simulink model "sigmadelta_full_DCO_Sampled_differential_integer_true"  (R2023b)
settings: Solver=VariableStepAuto  StartTime=0.0  StopTime=(lsim+10)*Ts  RelTol=1e-9
values from neighbouring files (symbols this model uses):
  f0 = fs*NC1/32    (= 98304000)    [exe_sigmadelta_full_DCO_differential_integer_true.m]
  f02 = f0    (= 98304000)    [exe_sigmadelta_full_DCO_differential_integer_true.m]
  ft = (bint-1)*fbin    [exe_sigmadelta_full_DCO_differential_integer_true.m]
  Input_signal = 10^(Input_signal_dB/20)    (= 0.24831331053)    [exe_sigmadelta_full_DCO_differential_integer_true.m]
  Kvco = f0*1    (= 98304000)    [exe_sigmadelta_full_DCO_differential_integer_true.m]
  NbC1 = Nbvco+Nbext    (= 10)    [exe_sigmadelta_full_DCO_differential_integer_true.m]
  Nbdcoext = 3    [exe_sigmadelta_full_DCO_differential_integer_true.m]
  T2 = 1/f2    (= 4.06901041667e-08)    [exe_sigmadelta_full_DCO_differential_integer_true.m]
  Ts = 1/fs    (= 3.25520833333e-07)    [exe_sigmadelta_full_DCO_differential_integer_true.m]
libraries: dspsigops x4
settings Model: SimulationMode=accelerator  ExtModeTrigDuration=100  Creator=user  LastModifiedBy=Richi
settings SolverCC: AlgebraicLoopSolver=TrustRegion
settings DataIOCC: SaveFinalState=on  SaveFormat=Array  SaveOutput=off  SaveState=on  ReturnWorkspaceOutputs=off  StateSaveName=tmp_raccel_xout  SignalLoggingName=tmp_raccel_logsout
settings OptimizationCC: BlockReduction=off  BooleanDataType=off  ReuseModelBlockBuffer=off  EfficientMapNaN2IntZero=off  LifeSpan=inf
settings DebuggingCC: SaveWithParameterizedLinksMsg=none  UnderspecifiedInitializationDetection=Classic  MergeDetectMultiDrivingBlocksExec=none  SignalResolutionControl=TryResolveAllWithWarning  MultiTaskDSMMsg=warning  MultiTaskCondExecSysMsg=none  UnconnectedInputMsg=warning  UnconnectedOutputMsg=warning  UnconnectedLineMsg=warning  SFUnexpectedBacktrackingDiag=warning  SFNoUnconditionalDefaultTransitionDiag=warning  SFExecutionAtInitializationDiag=none  ArithmeticOperatorsInVariantConditions=warning
settings HardwareCC: ProdBitPerPointer=32  ProdBitPerSizeT=32  ProdBitPerPtrDiffT=32  ProdLargestAtomicFloat=None  ProdIntDivRoundTo=Undefined  ProdEndianess=Unspecified  ProdWordSize=32  ProdHWDeviceType=32-bit Generic  TargetBitPerPointer=64  TargetBitPerSizeT=64  TargetBitPerPtrDiffT=64  TargetLongLongMode=on  TargetIntDivRoundTo=Zero  TargetEndianess=LittleEndian  TargetWordSize=64  TargetHWDeviceType=MATLAB Host  ProdEqTarget=off
settings ModelReferenceCC: EnableRefExpFcnMdlSchedulingChecks=on  PropagateSignalLabelsOutOfModel=off
settings SFSimCC: SimUseLocalCustomCode=off  CustomCodeUndefinedFunction=UseInterfaceOnly
settings RTWCC: SystemTargetFile=raccel.tlc  TemplateMakefile=raccel_default_tmf  RTWVerbose=off  RTWUseLocalCustomCode=off  RTWUseSimCustomCode=on  DLArmComputeVersion=19.05
settings CodeAppCC: GenerateComments=off  MaxIdLength=128  MangleLength=10  SimulinkBlockComments=off
settings RaccelTargetCC: ParMdlRefBuildCompliant=off  OptimizeReductions=off  ENABLE_SLEXEC_SSBRIDGE=0  RTWCAPISignals=off  RTWCAPIParams=off  RTWCAPIRootIO=off
settings ConfigComp: CovMetricSettings=dw  CovSaveCumulativeToWorkspaceVar=on  CovSaveSingleToWorkspaceVar=on  CovExternalEMLEnable=off

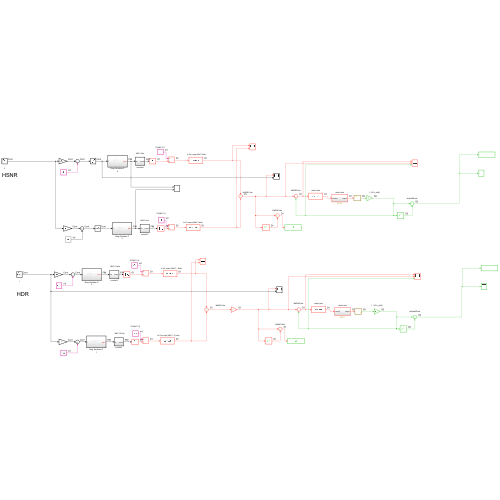
[thumbnail: Simulink's stored preview of the top-level diagram]
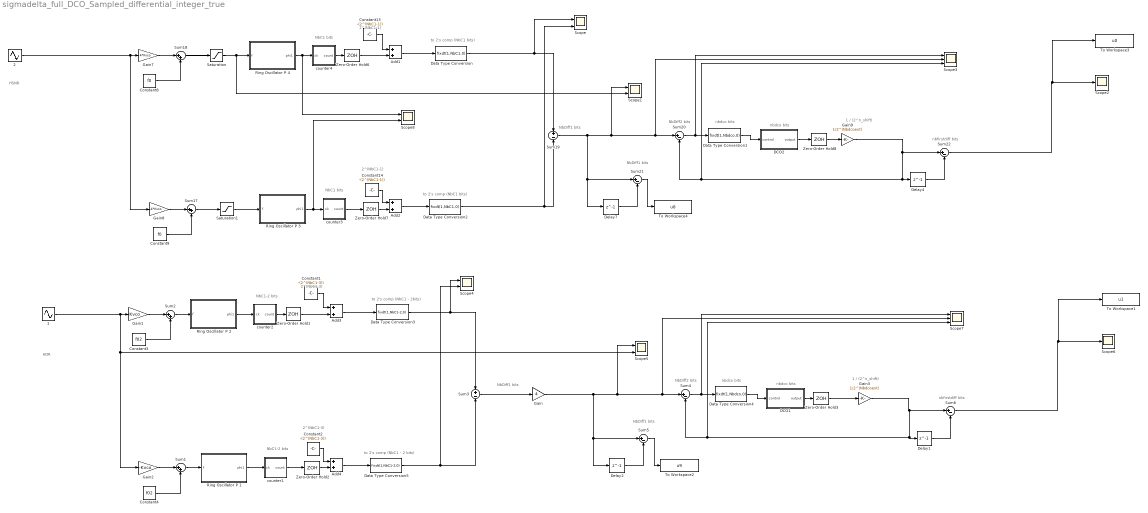
== system sigmadelta_full_DCO_Sampled_differential_integer_true ==
  note: HSNR
  note: nbfirstdiff bits
  note: 1 / (2^n_shift)
  note: nbdco bits
  note: NbDiff2 bits
  note: nbdco bits
  note: NbDiff1 bits
  note: 2^(NbC1-1)
  note: NbC1 bits
  note: NbC1 bits
  note: 2^(NbC1-1)
  note: to 2's comp (NbC1 bits)
  note: to 2's comp (NbC1 bits)
  note: NbDiff1 bits
  note: nbfirstdiff bits
  note: 1 / (2^n_shift)
  note: NbDiff1 bits
  note: to 2's comp (NbC1 - 2 bits)
  note: NbC1-2 bits
  note: nbdco bits
  note: NbDiff1 bits
  note: to 2's comp (NbC1 - 2bits)
  note: NbDiff2 bits
  note: NbC1-2 bits
  note: 2^(NbC1-3)
  note: nbdco bits
  note: 2^(NbC1-3)
  note: HDR
  " 1" : Sin  Amplitude=Input_signal  Frequency=2*pi*ft  SampleTime=0
  " 2" : Sin  Amplitude=Input_signal  Frequency=2*pi*ft  SampleTime=0
  Add{1..4} (4 alike) : Sum
  Constant1 : Constant  Value=-(2^(NbC1-3))
  Constant13 : Constant  Value=-(2^(NbC1-1))
  Constant14 : Constant  Value=-(2^(NbC1-1))
  Constant2 : Constant  Value=-(2^(NbC1-3))
  Constant3 : Constant  Value=f02
  Constant4 : Constant  Value=f02
  Constant8 : Constant  Value=f0
  Constant9 : Constant  Value=f0
  DCO1 : Subsystem
  DCO2 : Subsystem
  Data Type Conversion : DataTypeConversion  OutDataTypeStr=fixdt(1,NbC1,0)  SaturateOnIntegerOverflow=off  RndMeth=Floor
  Data Type Conversion1 : DataTypeConversion  OutDataTypeStr=fixdt(1,Nbdco,0)  SaturateOnIntegerOverflow=off  RndMeth=Floor
  Data Type Conversion2 : DataTypeConversion  OutDataTypeStr=fixdt(1,NbC1,0)  SaturateOnIntegerOverflow=off  RndMeth=Floor
  Data Type Conversion3 : DataTypeConversion  OutDataTypeStr=fixdt(1,NbC1-2,0)  SaturateOnIntegerOverflow=off  RndMeth=Floor
  Data Type Conversion4 : DataTypeConversion  OutDataTypeStr=fixdt(1,Nbdco,0)  SaturateOnIntegerOverflow=off  RndMeth=Floor
  Data Type Conversion5 : DataTypeConversion  OutDataTypeStr=fixdt(1,NbC1-2,0)  SaturateOnIntegerOverflow=off  RndMeth=Floor
  Delay1 : Delay  DelayLength=1  SampleTime=Ts
  Delay2 : Delay  DelayLength=1  SampleTime=T2
  Delay4 : Delay  DelayLength=1  SampleTime=Ts
  Delay7 : Delay  DelayLength=1  SampleTime=T2
  Gain : Gain  Gain=4  OutDataTypeStr=fixdt(1,NbDiff1,0)
  Gain1 : Gain  Gain=Kvco
  Gain2 : Gain  Gain=-Kvco
  Gain3 : Gain  Gain=1/2^(Nbdcoext)  OutDataTypeStr=fixdt(1,Nbvco+Nbext,0)
  Gain7 : Gain  Gain=4*Kvco
  Gain8 : Gain  Gain=-4*Kvco
  Gain9 : Gain  Gain=1/2^(Nbdcoext)  OutDataTypeStr=fixdt(1,Nbsd,0)
  Ring Oscillator P 1 : Subsystem
  Ring Oscillator P 2 : Subsystem
  Ring Oscillator P 3 : Subsystem
  Ring Oscillator P 4 : Subsystem
  Saturation : Saturate  UpperLimit=2*f0  LowerLimit=0
  Saturation1 : Saturate  UpperLimit=2*f0  LowerLimit=0
  Scope{,1,4..5,8} (5 alike) : Scope  NumInputPorts=2
  Scope2 : Scope
  Scope3 : Scope  NumInputPorts=3
  Scope6 : Scope
  Scope7 : Scope  NumInputPorts=3
  Sum{1..2,17..18} (4 alike) : Sum  Inputs=|++
  Sum19 : Sum  Inputs=+-  OutDataTypeStr=fixdt(1,NbDiff1,0)
  Sum20 : Sum  Inputs=|+-  OutDataTypeStr=fixdt(1,NbDiff2,0)
  Sum21 : Sum  Inputs=|+-  OutDataTypeStr=fixdt(1,NbDiff1,0)
  Sum22 : Sum  Inputs=|+-  OutDataTypeStr=fixdt(1,nbfirstdiff,0)
  Sum3 : Sum  Inputs=+-  OutDataTypeStr=fixdt(1,NbDiff1,0)
  Sum4 : Sum  Inputs=|+-  OutDataTypeStr=fixdt(1,NbDiff2,0)
  Sum5 : Sum  Inputs=|+-  OutDataTypeStr=fixdt(1,NbDiff1,0)
  Sum6 : Sum  Inputs=|+-  OutDataTypeStr=fixdt(1,nbfirstdiff,0)
  To Workspace1 : ToWorkspace  VariableName=u1  SampleTime=Ts
  To Workspace2 : ToWorkspace  VariableName=u9  SampleTime=Ts
  To Workspace3 : ToWorkspace  VariableName=u0  SampleTime=Ts
  To Workspace4 : ToWorkspace  VariableName=u8  SampleTime=Ts
  Zero-Order Hold{1..2,6..7} (4 alike) : ZeroOrderHold  SampleTime=T2
  Zero-Order Hold3 : ZeroOrderHold  SampleTime=Ts
  Zero-Order Hold8 : ZeroOrderHold  SampleTime=Ts
  counter1 : Subsystem
  counter2 : Subsystem
  counter3 : Subsystem
  counter4 : Subsystem
  wires:
  Constant9/1 -> Sum17/2
  Gain8/1 -> Sum17/1
  " 2"/1 -> Gain8/1, Gain7/1
  counter4/1(count) -> Zero-Order Hold6/1
  Ring Oscillator P 4/1(phi1) -> Scope8/1, counter4/1(ck)
  Sum17/1 -> Saturation1/1
  Sum18/1 -> Saturation/1
  Constant8/1 -> Sum18/2
  Gain7/1 -> Sum18/1
  Ring Oscillator P 3/1(phi1) -> Scope8/2, counter3/1(ck)
  counter3/1(count) -> Zero-Order Hold7/1
  Constant13/1 -> Add1/1
  Zero-Order Hold7/1 -> Add2/2
  Constant14/1 -> Add2/1
  Add1/1 -> Data Type Conversion/1
  Data Type Conversion/1 -> Scope/1, Sum19/1
  Add2/1 -> Data Type Conversion2/1
  Data Type Conversion2/1 -> Scope/2, Sum19/2
  Zero-Order Hold6/1 -> Add1/2
  Delay4/1 -> Sum22/2
  DCO2/1(output) -> Zero-Order Hold8/1
  Gain9/1 -> Scope3/3, Sum20/2, Delay4/1, Sum22/1
  Sum22/1 -> Scope2/1, To Workspace3/1
  Data Type Conversion1/1 -> DCO2/1(control)
  Zero-Order Hold8/1 -> Gain9/1
  Sum20/1 -> Scope3/1, Data Type Conversion1/1
  Sum19/1 -> Scope1/1, Scope3/2, Sum20/1, Sum21/1, Delay7/1
  Delay7/1 -> Sum21/2
  Sum21/1 -> To Workspace4/1
  Delay1/1 -> Sum6/2
  Sum5/1 -> To Workspace2/1
  Zero-Order Hold1/1 -> Add3/2
  Ring Oscillator P 2/1(phi1) -> counter2/1(ck)
  Sum2/1 -> Ring Oscillator P 2/1(f)
  counter2/1(count) -> Zero-Order Hold1/1
  Delay2/1 -> Sum5/2
  Sum1/1 -> Ring Oscillator P 1/1(f)
  Add4/1 -> Data Type Conversion5/1
  Ring Oscillator P 1/1(phi1) -> counter1/1(ck)
  Sum3/1 -> Gain/1
  Constant1/1 -> Add3/1
  Sum4/1 -> Scope7/1, Data Type Conversion4/1
  Zero-Order Hold3/1 -> Gain3/1
  Constant4/1 -> Sum1/2
  DCO1/1(output) -> Zero-Order Hold3/1
  Data Type Conversion4/1 -> DCO1/1(control)
  Data Type Conversion5/1 -> Sum3/2, Scope4/2
  Gain3/1 -> Scope7/3, Sum4/2, Delay1/1, Sum6/1
  Sum6/1 -> Scope6/1, To Workspace1/1
  Data Type Conversion3/1 -> Sum3/1, Scope4/1
  Gain1/1 -> Sum2/1
  Add3/1 -> Data Type Conversion3/1
  Constant3/1 -> Sum2/2
  " 1"/1 -> Gain2/1, Scope5/2, Gain1/1
  Zero-Order Hold2/1 -> Add4/2
  Gain2/1 -> Sum1/1
  counter1/1(count) -> Zero-Order Hold2/1
  Constant2/1 -> Add4/1
  Gain/1 -> Scope5/1, Scope7/2, Sum4/1, Sum5/1, Delay2/1
  Saturation/1 -> Scope1/2, Ring Oscillator P 4/1(f)
  Saturation1/1 -> Ring Oscillator P 3/1(f)

== system sigmadelta_full_DCO_Sampled_differential_integer_true/DCO1 ==
  control : Inport
  Delay2 : Delay  DelayLength=1  SampleTime=T2
  Sum2 : Sum  Inputs=|++  OutDataTypeStr=fixdt(1,Nbdco,0)
  Zero-Order Hold1 : ZeroOrderHold  SampleTime=T2
  output : Outport
  wires:
  Zero-Order Hold1/1 -> Delay2/1
  control/1 -> Sum2/1
  Sum2/1 -> Zero-Order Hold1/1
  Delay2/1 -> output/1, Sum2/2

== system sigmadelta_full_DCO_Sampled_differential_integer_true/DCO2 ==
  control : Inport
  Delay2 : Delay  DelayLength=1  SampleTime=T2
  Sum2 : Sum  Inputs=|++  OutDataTypeStr=fixdt(1,Nbdco,0)
  output : Outport
  wires:
  Sum2/1 -> Delay2/1
  control/1 -> Sum2/1
  Delay2/1 -> output/1, Sum2/2

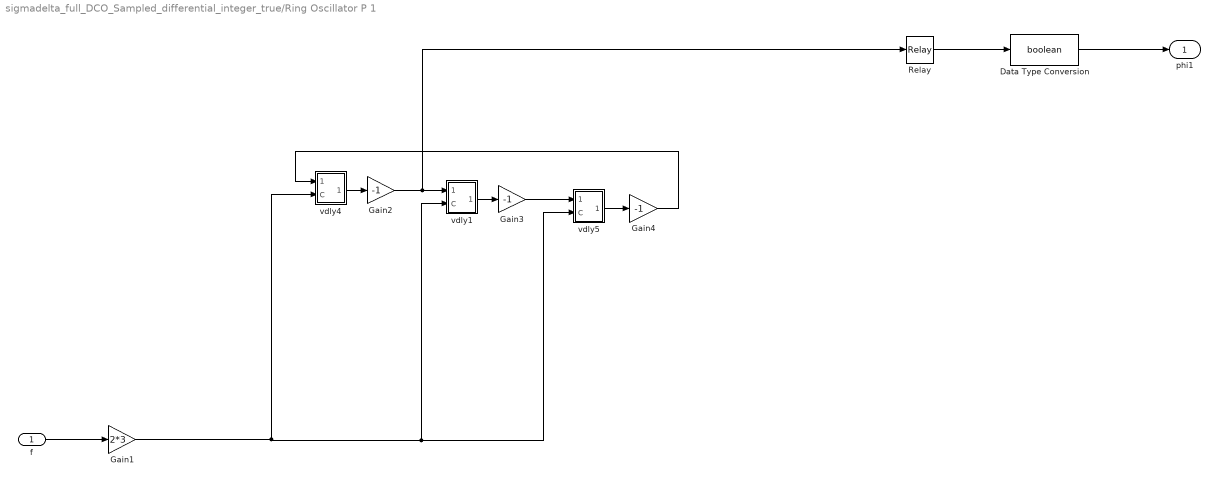
== system sigmadelta_full_DCO_Sampled_differential_integer_true/Ring Oscillator P 1 ==
  f : Inport
  Data Type Conversion : DataTypeConversion  OutDataTypeStr=boolean  SaturateOnIntegerOverflow=off  RndMeth=Floor
  Gain1 : Gain  Gain=2*3
  Gain2 : Gain  Gain=-1
  Gain3 : Gain  Gain=-1
  Gain4 : Gain  Gain=-1
  Relay : Relay
  vdly1 : Subsystem
  vdly4 : Subsystem
  vdly5 : Subsystem
  phi1 : Outport  VectorParamsAs1DForOutWhenUnconnected=off
  wires:
  vdly5/1(Out) -> Gain4/1
  vdly1/1(Out) -> Gain3/1
  vdly4/1(Out) -> Gain2/1
  f/1 -> Gain1/1
  Relay/1 -> Data Type Conversion/1
  Gain2/1 -> vdly1/1(In), Relay/1
  Gain3/1 -> vdly5/1(In)
  Data Type Conversion/1 -> phi1/1
  Gain1/1 -> vdly4/2(C), vdly1/2(C), vdly5/2(C)
  Gain4/1 -> vdly4/1(In)

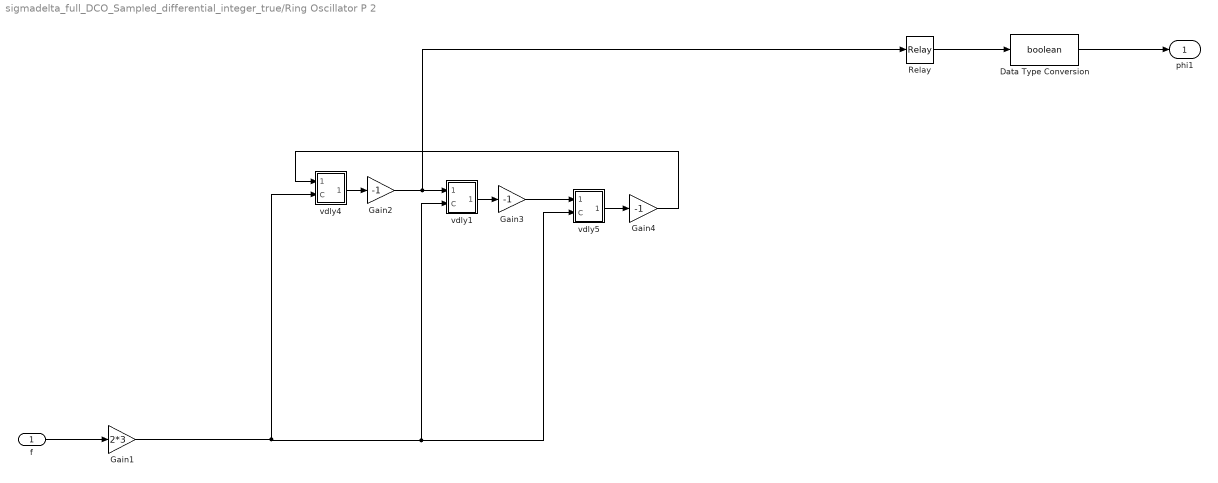
== system sigmadelta_full_DCO_Sampled_differential_integer_true/Ring Oscillator P 2 ==
  f : Inport
  Data Type Conversion : DataTypeConversion  OutDataTypeStr=boolean  SaturateOnIntegerOverflow=off  RndMeth=Floor
  Gain1 : Gain  Gain=2*3
  Gain2 : Gain  Gain=-1
  Gain3 : Gain  Gain=-1
  Gain4 : Gain  Gain=-1
  Relay : Relay
  vdly1 : Subsystem
  vdly4 : Subsystem
  vdly5 : Subsystem
  phi1 : Outport  VectorParamsAs1DForOutWhenUnconnected=off
  wires:
  vdly5/1(Out) -> Gain4/1
  vdly1/1(Out) -> Gain3/1
  vdly4/1(Out) -> Gain2/1
  f/1 -> Gain1/1
  Relay/1 -> Data Type Conversion/1
  Gain2/1 -> vdly1/1(In), Relay/1
  Gain3/1 -> vdly5/1(In)
  Data Type Conversion/1 -> phi1/1
  Gain1/1 -> vdly4/2(C), vdly1/2(C), vdly5/2(C)
  Gain4/1 -> vdly4/1(In)

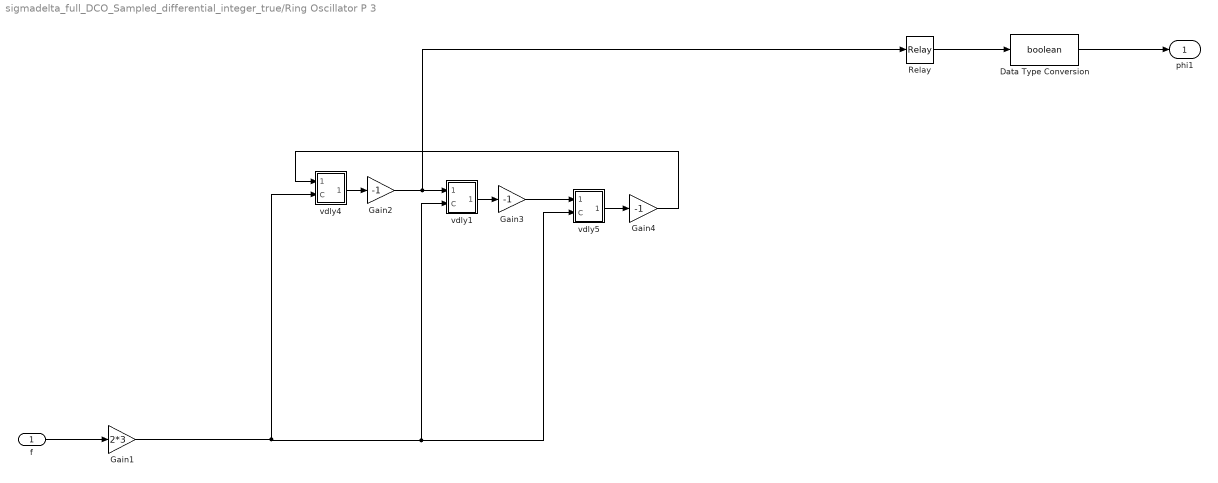
== system sigmadelta_full_DCO_Sampled_differential_integer_true/Ring Oscillator P 3 ==
  f : Inport
  Data Type Conversion : DataTypeConversion  OutDataTypeStr=boolean  SaturateOnIntegerOverflow=off  RndMeth=Floor
  Gain1 : Gain  Gain=2*3
  Gain2 : Gain  Gain=-1
  Gain3 : Gain  Gain=-1
  Gain4 : Gain  Gain=-1
  Relay : Relay
  vdly1 : Subsystem
  vdly4 : Subsystem
  vdly5 : Subsystem
  phi1 : Outport  VectorParamsAs1DForOutWhenUnconnected=off
  wires:
  vdly5/1(Out) -> Gain4/1
  vdly1/1(Out) -> Gain3/1
  vdly4/1(Out) -> Gain2/1
  f/1 -> Gain1/1
  Relay/1 -> Data Type Conversion/1
  Gain2/1 -> vdly1/1(In), Relay/1
  Gain3/1 -> vdly5/1(In)
  Data Type Conversion/1 -> phi1/1
  Gain1/1 -> vdly4/2(C), vdly1/2(C), vdly5/2(C)
  Gain4/1 -> vdly4/1(In)

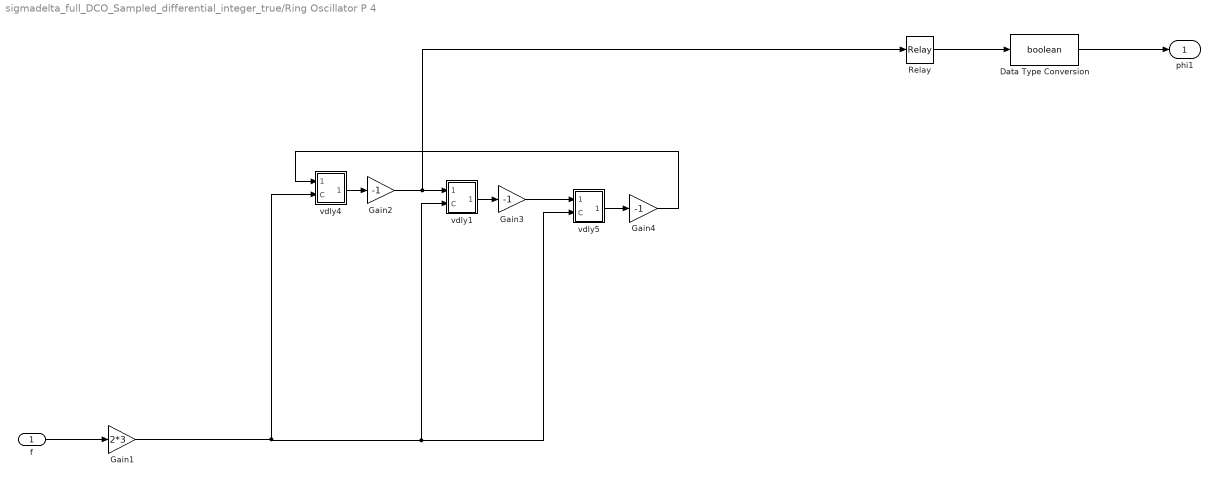
== system sigmadelta_full_DCO_Sampled_differential_integer_true/Ring Oscillator P 4 ==
  f : Inport
  Data Type Conversion : DataTypeConversion  OutDataTypeStr=boolean  SaturateOnIntegerOverflow=off  RndMeth=Floor
  Gain1 : Gain  Gain=2*3
  Gain2 : Gain  Gain=-1
  Gain3 : Gain  Gain=-1
  Gain4 : Gain  Gain=-1
  Relay : Relay
  vdly1 : Subsystem
  vdly4 : Subsystem
  vdly5 : Subsystem
  phi1 : Outport  VectorParamsAs1DForOutWhenUnconnected=off
  wires:
  vdly5/1(Out) -> Gain4/1
  vdly1/1(Out) -> Gain3/1
  vdly4/1(Out) -> Gain2/1
  f/1 -> Gain1/1
  Relay/1 -> Data Type Conversion/1
  Gain2/1 -> vdly1/1(In), Relay/1
  Gain3/1 -> vdly5/1(In)
  Data Type Conversion/1 -> phi1/1
  Gain1/1 -> vdly4/2(C), vdly1/2(C), vdly5/2(C)
  Gain4/1 -> vdly4/1(In)

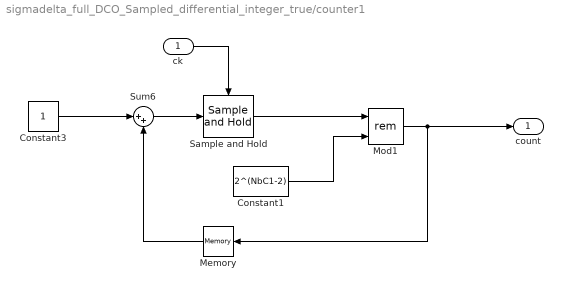
== system sigmadelta_full_DCO_Sampled_differential_integer_true/counter1 ==
  ck : Inport
  Constant1 : Constant  Value=2^(NbC1-2)
  Constant3 : Constant
  Memory : Memory
  Mod1 : Math  Operator=rem
  Sample and Hold : dspsigops/Sample and Hold  trig=Rising edge  initCond=0  latchinput=on
  Sum6 : Sum  Inputs=|++
  count : Outport
  wires:
  Constant3/1 -> Sum6/1
  Sum6/1 -> Sample and Hold/1
  ck/1 -> Sample and Hold/Trigger
  Memory/1 -> Sum6/2
  Constant1/1 -> Mod1/2
  Sample and Hold/1 -> Mod1/1
  Mod1/1 -> Memory/1, count/1

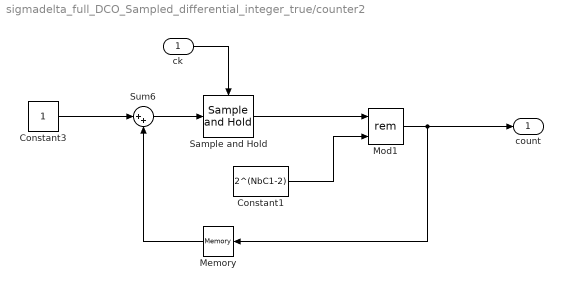
== system sigmadelta_full_DCO_Sampled_differential_integer_true/counter2 ==
  ck : Inport
  Constant1 : Constant  Value=2^(NbC1-2)
  Constant3 : Constant
  Memory : Memory
  Mod1 : Math  Operator=rem
  Sample and Hold : dspsigops/Sample and Hold  trig=Rising edge  initCond=0  latchinput=on
  Sum6 : Sum  Inputs=|++
  count : Outport
  wires:
  Constant3/1 -> Sum6/1
  Sum6/1 -> Sample and Hold/1
  ck/1 -> Sample and Hold/Trigger
  Memory/1 -> Sum6/2
  Constant1/1 -> Mod1/2
  Sample and Hold/1 -> Mod1/1
  Mod1/1 -> Memory/1, count/1

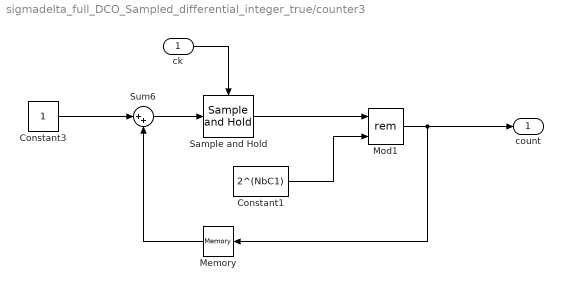
== system sigmadelta_full_DCO_Sampled_differential_integer_true/counter3 ==
  ck : Inport
  Constant1 : Constant  Value=2^(NbC1)
  Constant3 : Constant
  Memory : Memory
  Mod1 : Math  Operator=rem
  Sample and Hold : dspsigops/Sample and Hold  trig=Rising edge  initCond=0  latchinput=on
  Sum6 : Sum  Inputs=|++
  count : Outport
  wires:
  Constant3/1 -> Sum6/1
  Sum6/1 -> Sample and Hold/1
  ck/1 -> Sample and Hold/Trigger
  Memory/1 -> Sum6/2
  Constant1/1 -> Mod1/2
  Sample and Hold/1 -> Mod1/1
  Mod1/1 -> Memory/1, count/1

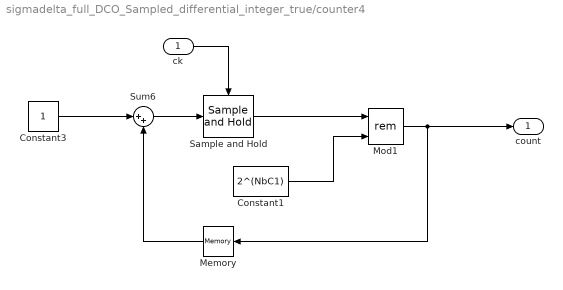
== system sigmadelta_full_DCO_Sampled_differential_integer_true/counter4 ==
  ck : Inport
  Constant1 : Constant  Value=2^(NbC1)
  Constant3 : Constant
  Memory : Memory
  Mod1 : Math  Operator=rem
  Sample and Hold : dspsigops/Sample and Hold  trig=Rising edge  initCond=0  latchinput=on
  Sum6 : Sum  Inputs=|++
  count : Outport
  wires:
  Constant3/1 -> Sum6/1
  Sum6/1 -> Sample and Hold/1
  ck/1 -> Sample and Hold/Trigger
  Memory/1 -> Sum6/2
  Constant1/1 -> Mod1/2
  Sample and Hold/1 -> Mod1/1
  Mod1/1 -> Memory/1, count/1

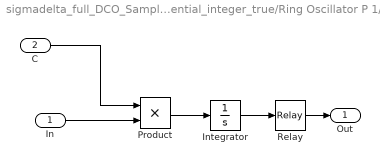
== system sigmadelta_full_DCO_Sampled_differential_integer_true/Ring Oscillator P 1/vdly1 ==
  In : Inport
  C : Inport  Port=2
  Integrator : Integrator  InitialCondition=-1  LimitOutput=on  UpperSaturationLimit=1  LowerSaturationLimit=-1
  Product : Product  RndMeth=Zero
  Relay : Relay  OffOutputValue=-1
  Out : Outport  VectorParamsAs1DForOutWhenUnconnected=off
  wires:
  Relay/1 -> Out/1
  Product/1 -> Integrator/1
  Integrator/1 -> Relay/1
  C/1 -> Product/1
  In/1 -> Product/2

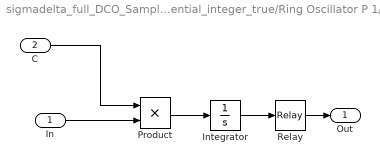
== system sigmadelta_full_DCO_Sampled_differential_integer_true/Ring Oscillator P 1/vdly4 ==
  In : Inport
  C : Inport  Port=2
  Integrator : Integrator  InitialCondition=1  LimitOutput=on  UpperSaturationLimit=1  LowerSaturationLimit=-1
  Product : Product  RndMeth=Zero
  Relay : Relay  OffOutputValue=-1
  Out : Outport  VectorParamsAs1DForOutWhenUnconnected=off
  wires:
  Relay/1 -> Out/1
  Product/1 -> Integrator/1
  Integrator/1 -> Relay/1
  C/1 -> Product/1
  In/1 -> Product/2

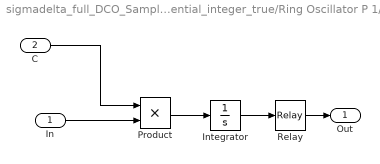
== system sigmadelta_full_DCO_Sampled_differential_integer_true/Ring Oscillator P 1/vdly5 ==
  In : Inport
  C : Inport  Port=2
  Integrator : Integrator  InitialCondition=-1  LimitOutput=on  UpperSaturationLimit=1  LowerSaturationLimit=-1
  Product : Product  RndMeth=Zero
  Relay : Relay  OffOutputValue=-1
  Out : Outport  VectorParamsAs1DForOutWhenUnconnected=off
  wires:
  Relay/1 -> Out/1
  Product/1 -> Integrator/1
  Integrator/1 -> Relay/1
  C/1 -> Product/1
  In/1 -> Product/2

== system sigmadelta_full_DCO_Sampled_differential_integer_true/Ring Oscillator P 2/vdly1 ==
  In : Inport
  C : Inport  Port=2
  Integrator : Integrator  InitialCondition=-1  LimitOutput=on  UpperSaturationLimit=1  LowerSaturationLimit=-1
  Product : Product  RndMeth=Zero
  Relay : Relay  OffOutputValue=-1
  Out : Outport  VectorParamsAs1DForOutWhenUnconnected=off
  wires:
  Relay/1 -> Out/1
  Product/1 -> Integrator/1
  Integrator/1 -> Relay/1
  C/1 -> Product/1
  In/1 -> Product/2

== system sigmadelta_full_DCO_Sampled_differential_integer_true/Ring Oscillator P 2/vdly4 ==
  In : Inport
  C : Inport  Port=2
  Integrator : Integrator  InitialCondition=1  LimitOutput=on  UpperSaturationLimit=1  LowerSaturationLimit=-1
  Product : Product  RndMeth=Zero
  Relay : Relay  OffOutputValue=-1
  Out : Outport  VectorParamsAs1DForOutWhenUnconnected=off
  wires:
  Relay/1 -> Out/1
  Product/1 -> Integrator/1
  Integrator/1 -> Relay/1
  C/1 -> Product/1
  In/1 -> Product/2

== system sigmadelta_full_DCO_Sampled_differential_integer_true/Ring Oscillator P 2/vdly5 ==
  In : Inport
  C : Inport  Port=2
  Integrator : Integrator  InitialCondition=-1  LimitOutput=on  UpperSaturationLimit=1  LowerSaturationLimit=-1
  Product : Product  RndMeth=Zero
  Relay : Relay  OffOutputValue=-1
  Out : Outport  VectorParamsAs1DForOutWhenUnconnected=off
  wires:
  Relay/1 -> Out/1
  Product/1 -> Integrator/1
  Integrator/1 -> Relay/1
  C/1 -> Product/1
  In/1 -> Product/2

== system sigmadelta_full_DCO_Sampled_differential_integer_true/Ring Oscillator P 3/vdly1 ==
  In : Inport
  C : Inport  Port=2
  Integrator : Integrator  InitialCondition=-1  LimitOutput=on  UpperSaturationLimit=1  LowerSaturationLimit=-1
  Product : Product  RndMeth=Zero
  Relay : Relay  OffOutputValue=-1
  Out : Outport  VectorParamsAs1DForOutWhenUnconnected=off
  wires:
  Relay/1 -> Out/1
  Product/1 -> Integrator/1
  Integrator/1 -> Relay/1
  C/1 -> Product/1
  In/1 -> Product/2

== system sigmadelta_full_DCO_Sampled_differential_integer_true/Ring Oscillator P 3/vdly4 ==
  In : Inport
  C : Inport  Port=2
  Integrator : Integrator  InitialCondition=1  LimitOutput=on  UpperSaturationLimit=1  LowerSaturationLimit=-1
  Product : Product  RndMeth=Zero
  Relay : Relay  OffOutputValue=-1
  Out : Outport  VectorParamsAs1DForOutWhenUnconnected=off
  wires:
  Relay/1 -> Out/1
  Product/1 -> Integrator/1
  Integrator/1 -> Relay/1
  C/1 -> Product/1
  In/1 -> Product/2

== system sigmadelta_full_DCO_Sampled_differential_integer_true/Ring Oscillator P 3/vdly5 ==
  In : Inport
  C : Inport  Port=2
  Integrator : Integrator  InitialCondition=-1  LimitOutput=on  UpperSaturationLimit=1  LowerSaturationLimit=-1
  Product : Product  RndMeth=Zero
  Relay : Relay  OffOutputValue=-1
  Out : Outport  VectorParamsAs1DForOutWhenUnconnected=off
  wires:
  Relay/1 -> Out/1
  Product/1 -> Integrator/1
  Integrator/1 -> Relay/1
  C/1 -> Product/1
  In/1 -> Product/2

== system sigmadelta_full_DCO_Sampled_differential_integer_true/Ring Oscillator P 4/vdly1 ==
  In : Inport
  C : Inport  Port=2
  Integrator : Integrator  InitialCondition=-1  LimitOutput=on  UpperSaturationLimit=1  LowerSaturationLimit=-1
  Product : Product  RndMeth=Zero
  Relay : Relay  OffOutputValue=-1
  Out : Outport  VectorParamsAs1DForOutWhenUnconnected=off
  wires:
  Relay/1 -> Out/1
  Product/1 -> Integrator/1
  Integrator/1 -> Relay/1
  C/1 -> Product/1
  In/1 -> Product/2

== system sigmadelta_full_DCO_Sampled_differential_integer_true/Ring Oscillator P 4/vdly4 ==
  In : Inport
  C : Inport  Port=2
  Integrator : Integrator  InitialCondition=1  LimitOutput=on  UpperSaturationLimit=1  LowerSaturationLimit=-1
  Product : Product  RndMeth=Zero
  Relay : Relay  OffOutputValue=-1
  Out : Outport  VectorParamsAs1DForOutWhenUnconnected=off
  wires:
  Relay/1 -> Out/1
  Product/1 -> Integrator/1
  Integrator/1 -> Relay/1
  C/1 -> Product/1
  In/1 -> Product/2

== system sigmadelta_full_DCO_Sampled_differential_integer_true/Ring Oscillator P 4/vdly5 ==
  In : Inport
  C : Inport  Port=2
  Integrator : Integrator  InitialCondition=-1  LimitOutput=on  UpperSaturationLimit=1  LowerSaturationLimit=-1
  Product : Product  RndMeth=Zero
  Relay : Relay  OffOutputValue=-1
  Out : Outport  VectorParamsAs1DForOutWhenUnconnected=off
  wires:
  Relay/1 -> Out/1
  Product/1 -> Integrator/1
  Integrator/1 -> Relay/1
  C/1 -> Product/1
  In/1 -> Product/2
